simulink model "Simulacion_diagrama_bloques"  (R2021a)
settings: Solver=VariableStepAuto  StartTime=0.0  StopTime=10.0  RelTol=1e-3
values from neighbouring files (symbols this model uses):
  k = 5    [Entregable_3.m]
settings Model: Creator=josef  LastModifiedBy=josef

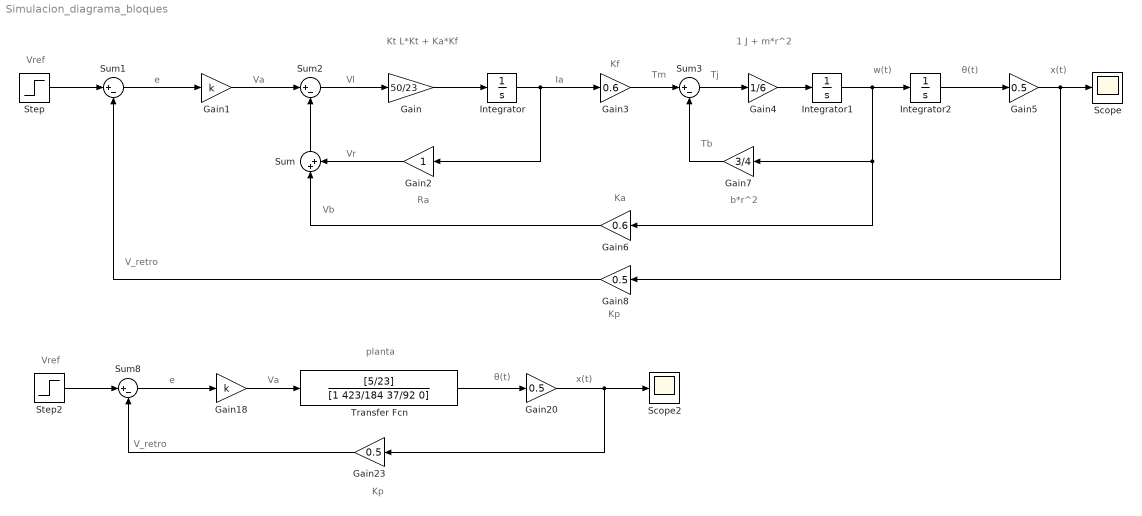
== system Simulacion_diagrama_bloques ==
  note: Vref
  note: e
  note: Va
  note: Vl
  note: Vr
  note: Vb
  note: Kt
      | L*Kt + Ka*Kf
  note: Ia
  note: Ra
  note: Kf
  note: Tm
  note: Tj
  note: 1
      | J + m*r^2
  note: Tb
  note: b*r^2
  note: w(t)
  note: θ(t)
  note: x(t)
  note: V_retro
  note: Ka
  note: x(t)
  note: Vref
  note: θ(t)
  note: Kp
  note: planta
  note: e
  note: Va
  note: V_retro
  note: Kp
  Gain : Gain  Gain=50/23
  Gain1 : Gain  Gain=k
  Gain18 : Gain  Gain=k
  Gain2 : Gain
  Gain{5,8,20,23} (4 alike) : Gain  Gain=0.5
  Gain3 : Gain  Gain=0.6
  Gain4 : Gain  Gain=1/6
  Gain6 : Gain  Gain=0.6
  Gain7 : Gain  Gain=3/4
  Integrator : Integrator
  Integrator1 : Integrator
  Integrator2 : Integrator
  Scope : Scope
  Scope2 : Scope
  Step : Step  SampleTime=0
  Step2 : Step  SampleTime=0
  Sum : Sum  Inputs=|++
  Sum{1..3,8} (4 alike) : Sum  Inputs=|+-
  Transfer Fcn : TransferFcn  Numerator=[5/23]  Denominator=[1 423/184 37/92 0]
  wires:
  Step/1 -> Sum1/1
  Sum1/1 -> Gain1/1
  Gain1/1 -> Sum2/1
  Sum/1 -> Sum2/2
  Sum2/1 -> Gain/1
  Gain/1 -> Integrator/1
  Gain2/1 -> Sum/2
  Integrator/1 -> Gain3/1, Gain2/1
  Gain3/1 -> Sum3/1
  Sum3/1 -> Gain4/1
  Gain4/1 -> Integrator1/1
  Integrator1/1 -> Gain7/1, Gain6/1, Integrator2/1
  Integrator2/1 -> Gain5/1
  Gain5/1 -> Gain8/1, Scope/1
  Gain6/1 -> Sum/1
  Gain7/1 -> Sum3/2
  Gain8/1 -> Sum1/2
  Sum8/1 -> Gain18/1
  Gain18/1 -> Transfer Fcn/1
  Transfer Fcn/1 -> Gain20/1
  Gain20/1 -> Scope2/1, Gain23/1
  Step2/1 -> Sum8/1
  Gain23/1 -> Sum8/2
